simulink library "INT_FuelConsDspl_DD"  (R2016b)
settings: Solver=VariableStepAuto  StartTime=0.0  StopTime=10.0  RelTol=1e-3
settings Model: Creator=liutao  LastModifiedBy=liutao

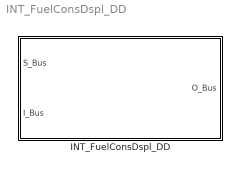
== system INT_FuelConsDspl_DD ==
  INT_FuelConsDspl_DD : Subsystem

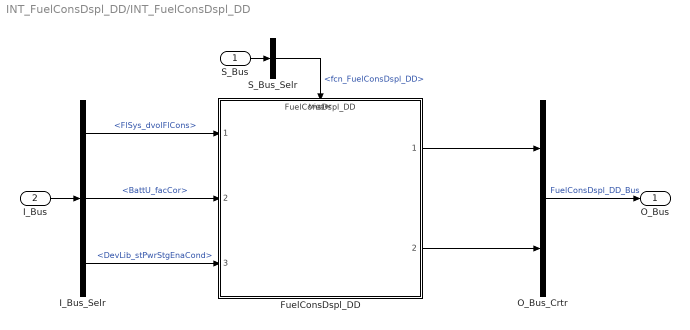
== system INT_FuelConsDspl_DD/INT_FuelConsDspl_DD ==
  S_Bus : Inport
  I_Bus : Inport  Port=2
  FuelConsDspl_DD : ModelReference  ModelNameDialog=FuelConsDspl_DD  SimulationMode=Normal  ModelReferenceVersion=1.15  TriggerPortName=function  TriggerPortTriggerType=function-call  TriggerPortStatesWhenEnabling=held
  I_Bus_Selr : BusSelector  OutputSignals=FlSys_dvolFlCons,BattU_facCor,DevLib_stPwrStgEnaCond
  O_Bus_Crtr : BusCreator  Inputs=2
  S_Bus_Selr : BusSelector  OutputSignals=fcn_FuelConsDspl_DD
  O_Bus : Outport
  wires:
  S_Bus_Selr/1 -> FuelConsDspl_DD/Trigger  "<fcn_FuelConsDspl_DD>"
  S_Bus/1 -> S_Bus_Selr/1
  I_Bus/1 -> I_Bus_Selr/1
  I_Bus_Selr/1 -> FuelConsDspl_DD/1  "<FlSys_dvolFlCons>"
  I_Bus_Selr/2 -> FuelConsDspl_DD/2  "<BattU_facCor>"
  I_Bus_Selr/3 -> FuelConsDspl_DD/3  "<DevLib_stPwrStgEnaCond>"
  O_Bus_Crtr/1 -> O_Bus/1  "FuelConsDspl_DD_Bus"
  FuelConsDspl_DD/1 -> O_Bus_Crtr/1
  FuelConsDspl_DD/2 -> O_Bus_Crtr/2
